simulink model "seldom_sim"  (R2024a)
settings: Solver=FixedStepAuto  StartTime=0.0  StopTime=30  FixedStep=framePeriod_s  RelTol=1e-9
values from neighbouring files (symbols this model uses):
  framePeriod_s = 1/frameRate_hz    (= 0.02)    [setup.m]
undefined symbols (not defined in the file or in its folder): accel_mps2, Aircraft, alt_wgs84_m, ch, current_ma, datetime, datevec, die_temp_c, Earth, Env, ext_gnss1, failsafe, fmu_imu, fmu_mag, frame_time_us, gps_tow_ms, gyro_radps, healthy, horz_acc_m, imu_healthy, inceptor, InitCond, installed, lat_rad, lon_rad, lost_frame, mag_ut, ned_vel_mps, new_data, num_sats, power_module, sys_time_us, Telem, vert_acc_m, voltage_v, week, WGS84
libraries: simulink x8, aerolibconvert2 x5, aerolibasang x3, aerolibtransform2 x2, aerolibgravity2 x2, aerolibatmos2 x1, sharedtransform x1, uavutilslib x1, vrlib x1, simulink_extras x1, spsLeadLagFilterLib x1, shared6dof x1
(part 1 of 2)
settings Model: SILPILSystemUnderTest=refmodels  Creator=brian  LastModifiedBy=joshb
settings SolverCC: AlgebraicLoopSolver=TrustRegion
settings DataIOCC: SaveOutput=off  SignalLogging=off  DSMLogging=off  SaveTime=off  ReturnWorkspaceOutputsName=Data
settings OptimizationCC: DefaultParameterBehavior=Inlined  EnhancedBackFolding=on  PassReuseOutputArgsAs=Individual arguments  ZeroExternalMemoryAtStartup=off  ZeroInternalMemoryAtStartup=off  OptimizeBlockOrder=speed  DifferentSizesBufferReuse=on  EfficientTunableParamExpr=on
settings DebuggingCC: Int32ToFloatConvMsg=none  ParameterPrecisionLossMsg=none  ParameterTunabilityLossMsg=error  UnconnectedInputMsg=warning  UnconnectedOutputMsg=warning  UnconnectedLineMsg=warning
settings HardwareCC: ProdBitPerPointer=32  ProdBitPerSizeT=32  ProdBitPerPtrDiffT=32  ProdLargestAtomicInteger=Long  ProdLargestAtomicFloat=Double  ProdWordSize=32  ProdHWDeviceType=NXP->Cortex-M4  TargetBitPerLong=64  TargetBitPerPointer=64  TargetBitPerSizeT=64  TargetBitPerPtrDiffT=64  TargetLargestAtomicFloat=Float  TargetIntDivRoundTo=Zero  TargetEndianess=LittleEndian  TargetWordSize=64  TargetHWDeviceType=Intel->x86-64 (Linux 64)  ProdEqTarget=off
settings ModelReferenceCC: UpdateModelReferenceTargets=Force  EnableRefExpFcnMdlSchedulingChecks=on
settings SFSimCC: SimCustomCompilerFlags=-std=c++2a, -fconcepts, -felide-constructors  SimCustomLinkerFlags=-std=c++2a, -fconcepts, -felide-constructors  MATLABDynamicMemAlloc=off  SimTargetLang=C++
settings RTWCC: Description=Embedded Coder  SystemTargetFile=ert.tlc  GenCodeOnly=on  TemplateMakefile=ert_default_tmf  RTWUseSimCustomCode=on  TargetLang=C++  GPUComputeCapability=3.5  DLArmComputeVersion=19.05
settings CodeAppCC: ForceParamTrailComments=on  IgnoreCustomStorageClasses=off  OperatorAnnotations=on  SimulinkDataObjDesc=on  SFDataObjDesc=on  InsertBlockDesc=on
settings ERTTargetCC: TargetLangStandard=C++11 (ISO)  GenerateSampleERTMain=on  CodeInterfacePackaging=C++ class  InlinedParameterPlacement=NonHierarchical  RootIOFormat=Structure reference  ERTCustomFileTemplate=example_file_process.tlc

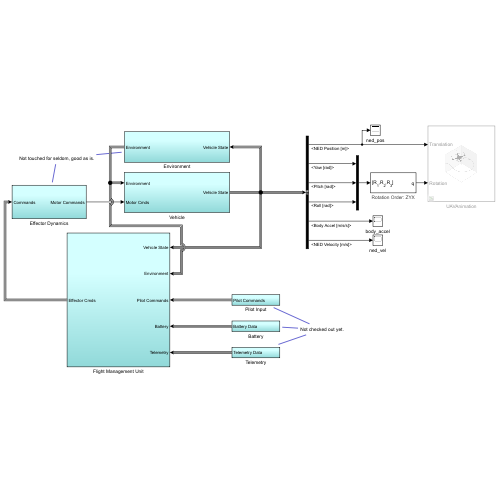
[thumbnail: Simulink's stored preview of the top-level diagram]
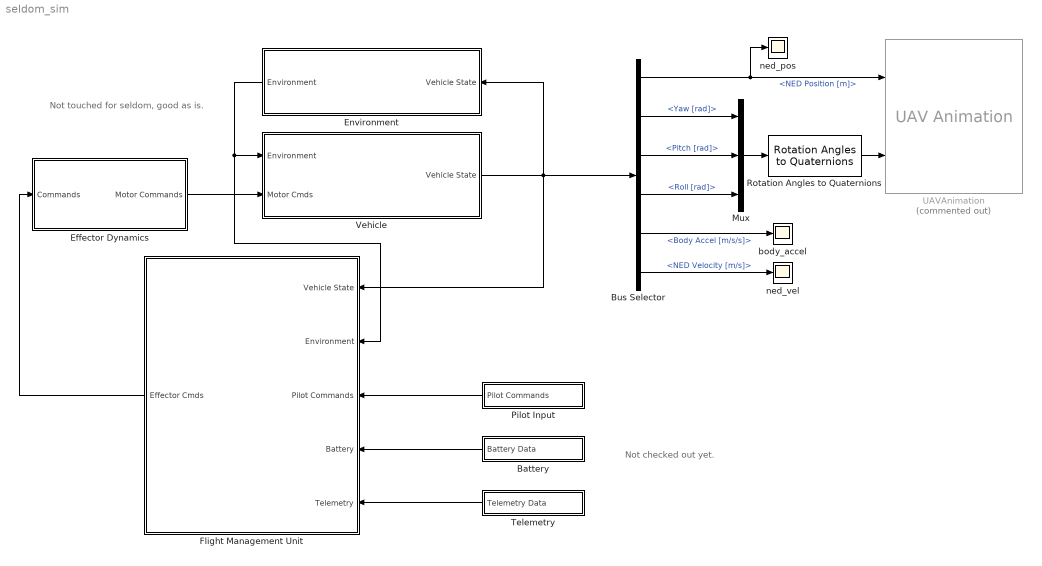
== system seldom_sim ==
  note: Not touched for seldom, good as is.
  note: Not checked out yet.
  Battery : Subsystem
  Bus Selector : BusSelector  OutputSignals=NED Position [m],Yaw [rad],Pitch [rad],Roll [rad],Body Accel [m/s/s],NED Velocity [m/s]
  Effector Dynamics : Subsystem
  Environment : Subsystem
  Flight Management Unit : Subsystem
  Mux : Mux  Inputs=3
  Pilot Input : Subsystem
  Rotation Angles to Quaternions : sharedtransform/Rotation Angles to Quaternions  rotationOrder=ZYX  aMode=aMode
  Telemetry : Subsystem
  UAVAnimation : uavutilslib/UAV Animation  Commented=on  UAVType=Multirotor  UAVSize=1  InertialZDirection=Down  SampleTime=-1
  Vehicle : Subsystem
  body_accel : Scope
  ned_pos : Scope
  ned_vel : Scope
  wires:
  Vehicle/1(Vehicle State) -> Environment/1(Vehicle State), Bus Selector/1, Flight Management Unit/1(Vehicle State)
  Pilot Input/1(Pilot Commands) -> Flight Management Unit/3(Pilot Commands)
  Environment/1(Environment) -> Vehicle/1(Environment), Flight Management Unit/2(Environment)
  Effector Dynamics/1(Motor Commands) -> Vehicle/2(Motor Cmds)
  Telemetry/1(Telemetry Data) -> Flight Management Unit/5(Telemetry)
  Flight Management Unit/1(Effector Cmds) -> Effector Dynamics/1(Commands)
  Battery/1(Battery Data) -> Flight Management Unit/4(Battery)
  Bus Selector/1 -> UAVAnimation/1, ned_pos/1  "<NED Position [m]>"
  Bus Selector/4 -> Mux/3  "<Roll [rad]>"
  Bus Selector/2 -> Mux/1  "<Yaw [rad]>"
  Bus Selector/3 -> Mux/2  "<Pitch [rad]>"
  Mux/1 -> Rotation Angles to Quaternions/1
  Rotation Angles to Quaternions/1 -> UAVAnimation/2
  Bus Selector/5 -> body_accel/1  "<Body Accel [m/s/s]>"
  Bus Selector/6 -> ned_vel/1  "<NED Velocity [m/s]>"

== system seldom_sim/Battery ==
  note: All of this needs updated for seldom. Or more likely it can all just go away, probably don't need it.
  note: This is the amp draw from the battery
  note: The mRo Power Zero module
      | outputs 1V for 33.594 amps drawn
      | from the battery
  note: This is the voltage measured by the FMU
      | power port. It is typically the current, scaled
      | by the power module mA / volt
  note: This is the voltage
      | measured by the FMU at
      | the power port. It is typically
      | the battery voltage scaled by the
      | power module voltage divider.
  note: The mRo Power Zero module
      | outputs 1V for 15.30 V at the
      | battery
  Bus Creator : BusCreator  Inputs=2
  Cast To Single : DataTypeConversion  OutDataTypeStr=single  SaturateOnIntegerOverflow=off  RndMeth=Floor
  Cast To Single1 : DataTypeConversion  OutDataTypeStr=single  SaturateOnIntegerOverflow=off  RndMeth=Floor
  Constant : Constant  Value=Aircraft.Battery.Voltage
  Constant1 : Constant  Value=42
  Constant2 : Constant
  Constant3 : Constant
  Divide : Product  Inputs=*/
  Divide1 : Product  Inputs=*/
  Battery Data : Outport
  wires:
  Bus Creator/1 -> Battery Data/1
  Constant2/1 -> Divide/2
  Constant1/1 -> Divide/1
  Divide/1 -> Cast To Single1/1  "Current [V]"
  Divide1/1 -> Cast To Single/1  "Voltage [V]"
  Constant/1 -> Divide1/1
  Constant3/1 -> Divide1/2
  Cast To Single/1 -> Bus Creator/1  "Voltage [V]"
  Cast To Single1/1 -> Bus Creator/2  "Current [V]"

== system seldom_sim/Effector Dynamics ==
  Commands : Inport
  Add1 : Sum
  Bus Selector : BusSelector  OutputSignals=pwm
  Constant : Constant  Value=0
  Constant1 : Constant  Commented=on  Value=InitCond.motor_cmd
  Selector1 : Selector  InputPortWidth=Aircraft.Eff.nPwm  IndexOptions=Index vector (dialog)  Indices=Aircraft.Motor.map  OutputSizes=1
  Motor Commands : Outport
  wires:
  Constant/1 -> Add1/2
  Selector1/1 -> Add1/1
  Bus Selector/1 -> Selector1/1  "<pwm>"
  Commands/1 -> Bus Selector/1
  Add1/1 -> Motor Commands/1

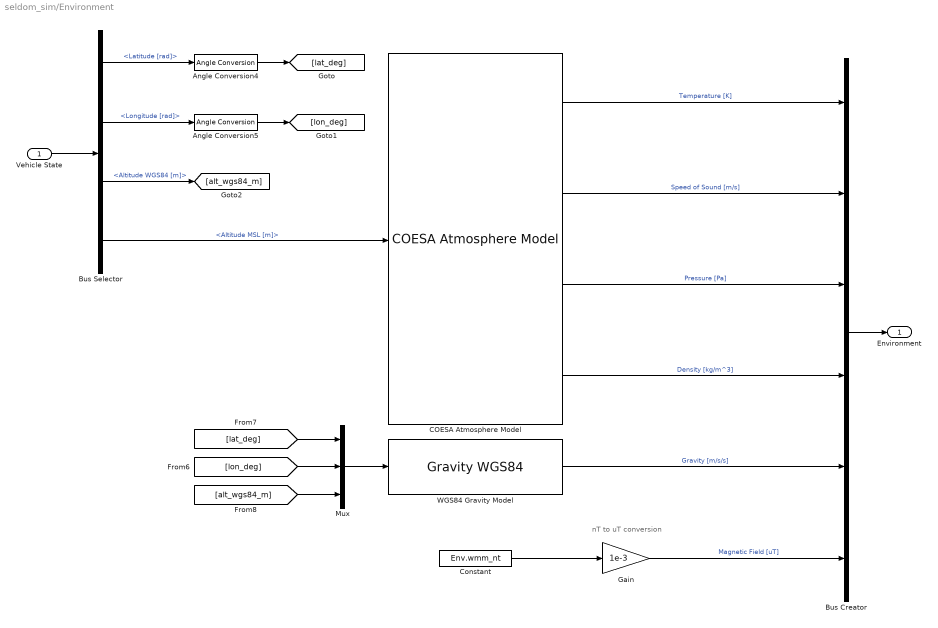
== system seldom_sim/Environment ==
  note: nT to uT conversion
  Vehicle State : Inport
  Angle Conversion4 : aerolibconvert2/Angle Conversion  IU=rad  OU=deg
  Angle Conversion5 : aerolibconvert2/Angle Conversion  IU=rad  OU=deg
  Bus Creator : BusCreator  Inputs=6
  Bus Selector : BusSelector  OutputSignals=Latitude [rad],Longitude [rad],Altitude WGS84 [m],Altitude MSL [m]
  COESA Atmosphere Model : aerolibatmos2/COESA Atmosphere Model  units=Metric (MKS)  spec=1976 COESA-extended U.S. Standard Atmosphere  model=Profile  profile_var=High temperature  profile_percent=1%  profile_alt=5 km (16404 ft)  envelope_var=High temperature  envelope_percent=1%  action=Warning
  Constant : Constant  Value=Env.wmm_nt
  Gain : Gain  Gain=1e-3
  Mux : Mux  Inputs=3
  "WGS84 Gravity Model  " : GravityWGS84
  Environment : Outport
  wires:
  [lon_deg] -> Mux/2
  COESA Atmosphere Model/4 -> Bus Creator/4  "Density [kg/m^3]"
  Mux/1 -> "WGS84 Gravity Model  "/1
  Bus Selector/3 -> [alt_wgs84_m]  "<Altitude WGS84 [m]>"
  Vehicle State/1 -> Bus Selector/1
  Bus Selector/2 -> Angle Conversion5/1  "<Longitude [rad]>"
  COESA Atmosphere Model/2 -> Bus Creator/2  "Speed of Sound [m/s]"
  Bus Selector/4 -> COESA Atmosphere Model/1  "<Altitude MSL [m]>"
  [alt_wgs84_m] -> Mux/3
  Angle Conversion4/1 -> [lat_deg]
  [lat_deg] -> Mux/1
  Bus Creator/1 -> Environment/1
  Constant/1 -> Gain/1
  Gain/1 -> Bus Creator/6  "Magnetic Field [uT]"
  "WGS84 Gravity Model  "/1 -> Bus Creator/5  "Gravity [m/s/s]"
  Bus Selector/1 -> Angle Conversion4/1  "<Latitude [rad]>"
  COESA Atmosphere Model/3 -> Bus Creator/3  "Pressure [Pa]"
  COESA Atmosphere Model/1 -> Bus Creator/1  "Temperature [K]"
  Angle Conversion5/1 -> [lon_deg]

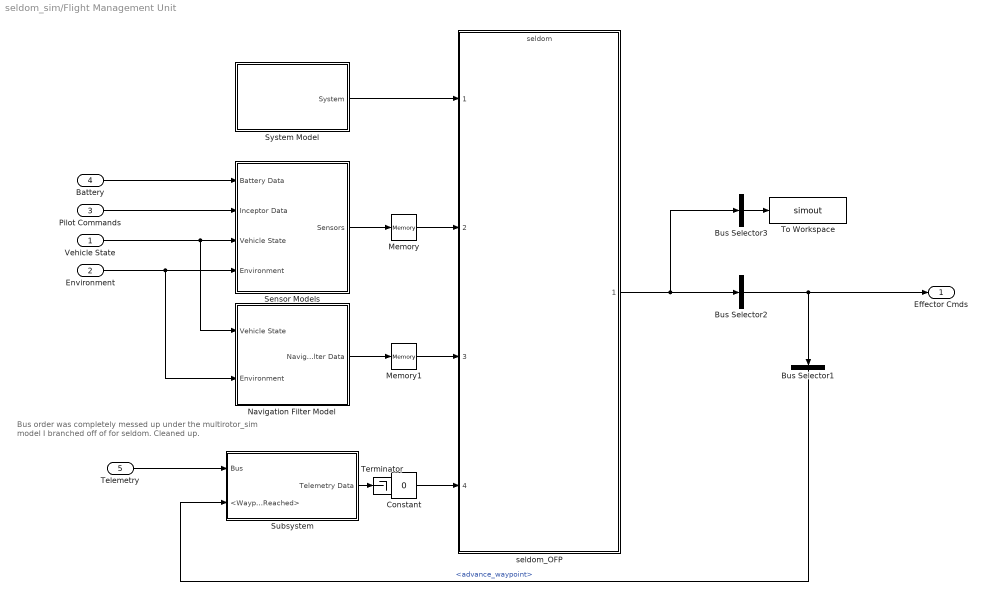
== system seldom_sim/Flight Management Unit ==
  note: Bus order was completely messed up under the multirotor_sim model I branched off of for seldom. Cleaned up.
  Vehicle State : Inport
  Environment : Inport  Port=2
  Pilot Commands : Inport  Port=3
  Battery : Inport  Port=4
  Telemetry : Inport  Port=5
  Bus Selector1 : BusSelector  OutputSignals=advance_waypoint
  Bus Selector2 : BusSelector  OutputSignals=advance_waypoint,sbus,pwm  OutputAsBus=on
  Bus Selector3 : BusSelector  OutputSignals=aux  OutputAsBus=on
  Constant : Constant  Value=0  OutDataTypeStr=Bus: TelemData
  Memory : Memory  InheritSampleTime=on  LinearizeMemory=on  LinearizeAsDelay=on
  Memory1 : Memory  InheritSampleTime=on  LinearizeMemory=on  LinearizeAsDelay=on
  Navigation Filter Model : Subsystem
      settings: PortSchema="{\"entries\":[{\"content\":{\"sides\":[{\"content\":{\"connectorIds\":[]},\"type\":\"ConnectorPlacement.EquallySpacedRectSide\",\"uuid\":\"b20f7590-d69b-48b8-beb1-2fb7d3ab0357\"},{\"content\":{\"connectorIds\":[],\"side\":\"RIGHT\"},\"type\":\"ConnectorPlacement.EquallySpacedRectSide\",\"uuid\":\"07801f8a-7756-483e-a050-3c2fccc33404\"},{\"content\":{\"connectorIds\":[\"In1\",\"In2\"],\"side\":\"TOP\"},\"type\":\"ConnectorPlacement.EquallySpacedRectSide\",\"uuid\":\"ce3c3c94-ed36-4103-b079-69dcaeaf21e9\"},{\"content\":{\"connectorIds\":[\"Out1\"],\"side\":\"BOTTOM\"},\"type\":\"ConnectorPlacement.EquallySpacedRectSide\",\"uuid\":\"ba78b819-a471-4bc3-b479-e6a973cfe14f\"},{\"content\":{\"connectorIds\":[],\"side\":\"HIDDEN\"},\"type\":\"ConnectorPlacement.EquallySpacedRectSide\",\"uuid\":\"3cf915a5-25a1-4380-9090-9561533312da\"}]},\"type\":\"ConnectorPlacement.EquallySpacedConnector\",\"uuid\":\"7ef4ddaa-ccd2-4778-89ce-8b4685524e82\"}],\"packageUris\":[\"http://schema.mathworks.com/mf0/Connector/R2020b\"],\"version\":\"1.0\"}"
  Sensor Models : Subsystem
      settings: PortSchema="{\"entries\":[{\"content\":{\"sides\":[{\"content\":{},\"type\":\"ConnectorPlacement.EquallySpacedRectSide\",\"uuid\":\"b20f7590-d69b-48b8-beb1-2fb7d3ab0357\"},{\"content\":{\"side\":\"RIGHT\"},\"type\":\"ConnectorPlacement.EquallySpacedRectSide\",\"uuid\":\"07801f8a-7756-483e-a050-3c2fccc33404\"},{\"content\":{\"connectorIds\":[\"In1\",\"In2\",\"In3\",\"In4\"],\"side\":\"TOP\"},\"type\":\"ConnectorPlacement.EquallySpacedRectSide\",\"uuid\":\"ce3c3c94-ed36-4103-b079-69dcaeaf21e9\"},{\"content\":{\"connectorIds\":[\"Out1\"],\"side\":\"BOTTOM\"},\"type\":\"ConnectorPlacement.EquallySpacedRectSide\",\"uuid\":\"ba78b819-a471-4bc3-b479-e6a973cfe14f\"},{\"content\":{\"side\":\"HIDDEN\"},\"type\":\"ConnectorPlacement.EquallySpacedRectSide\",\"uuid\":\"3cf915a5-25a1-4380-9090-9561533312da\"}]},\"type\":\"ConnectorPlacement.EquallySpacedConnector\",\"uuid\":\"7ef4ddaa-ccd2-4778-89ce-8b4685524e82\"}],\"packageUris\":[\"http://schema.mathworks.com/mf0/Connector/R2020b\"],\"version\":\"1.0\"}"
  Subsystem : Subsystem
  System Model : Subsystem
      settings: PortSchema="{\"entries\":[{\"content\":{\"sides\":[{\"content\":{\"connectorIds\":[]},\"type\":\"ConnectorPlacement.EquallySpacedRectSide\",\"uuid\":\"b20f7590-d69b-48b8-beb1-2fb7d3ab0357\"},{\"content\":{\"connectorIds\":[],\"side\":\"RIGHT\"},\"type\":\"ConnectorPlacement.EquallySpacedRectSide\",\"uuid\":\"07801f8a-7756-483e-a050-3c2fccc33404\"},{\"content\":{\"connectorIds\":[],\"side\":\"TOP\"},\"type\":\"ConnectorPlacement.EquallySpacedRectSide\",\"uuid\":\"ce3c3c94-ed36-4103-b079-69dcaeaf21e9\"},{\"content\":{\"connectorIds\":[\"Out1\"],\"side\":\"BOTTOM\"},\"type\":\"ConnectorPlacement.EquallySpacedRectSide\",\"uuid\":\"ba78b819-a471-4bc3-b479-e6a973cfe14f\"},{\"content\":{\"connectorIds\":[],\"side\":\"HIDDEN\"},\"type\":\"ConnectorPlacement.EquallySpacedRectSide\",\"uuid\":\"3cf915a5-25a1-4380-9090-9561533312da\"}]},\"type\":\"ConnectorPlacement.EquallySpacedConnector\",\"uuid\":\"7ef4ddaa-ccd2-4778-89ce-8b4685524e82\"}],\"packageUris\":[\"http://schema.mathworks.com/mf0/Connector/R2020b\"],\"version\":\"1.0\"}"
  Terminator : Terminator
  To Workspace : ToWorkspace  VariableName=simout  SaveFormat=Timeseries  SampleTime=-1
  seldom_OFP : ModelReference  ModelNameDialog=seldom.slx  SimulationMode=Normal  ModelReferenceVersion=8.65
  Effector Cmds : Outport
  wires:
  Environment/1 -> Navigation Filter Model/1(Environment), Sensor Models/1(Environment)
  Vehicle State/1 -> Navigation Filter Model/2(Vehicle State), Sensor Models/2(Vehicle State)
  Sensor Models/1(Sensors) -> Memory/1
  Navigation Filter Model/1(Navigation Filter Data) -> Memory1/1
  System Model/1(System) -> seldom_OFP/1
  Pilot Commands/1 -> Sensor Models/3(Inceptor Data)
  Telemetry/1 -> Subsystem/1(Bus)
  Memory/1 -> seldom_OFP/2
  Memory1/1 -> seldom_OFP/3
  Battery/1 -> Sensor Models/4(Battery Data)
  Subsystem/1(Telemetry Data) -> Terminator/1
  Bus Selector1/1 -> Subsystem/2(<Waypoint Reached>)  "<advance_waypoint>"
  Bus Selector2/1 -> Bus Selector1/1, Effector Cmds/1
  seldom_OFP/1 -> Bus Selector3/1, Bus Selector2/1
  Constant/1 -> seldom_OFP/4
  Bus Selector3/1 -> To Workspace/1

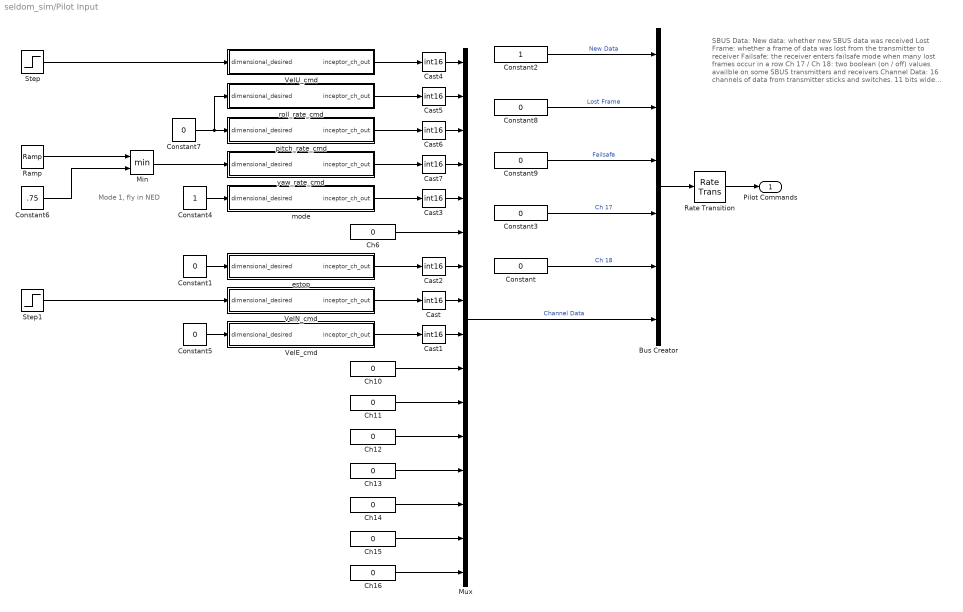
== system seldom_sim/Pilot Input ==
  note: Mode 1, fly in NED
  note: SBUS Data:
      | New data: whether new SBUS data was received
      | Lost Frame: whether a frame of data was lost from the transmitter to receiver
      | Failsafe: the receiver enters failsafe mode when many lost frames occur in a row
      | Ch 17 / Ch 18: two boolean (on / off) values availble on some SBUS transmitters and receivers
      | Channel Data: 16 channels of data from transmitter sticks and switches. 11 bits wide limiting values to 0 - 2048. Actual ranges may be different, for example, FrSky typically uses 172 - 1811 unless its range is extended to +/- 150%
  Bus Creator : BusCreator  Inputs=6
  Cast{,1..7} (8 alike) : DataTypeConversion  OutDataTypeStr=int16  SaturateOnIntegerOverflow=off  RndMeth=Floor
  Ch{6,10..16} (8 alike) : Constant  Value=0  OutDataTypeStr=int16
  Constant : Constant  Value=0  OutDataTypeStr=int8
  Constant1 : Constant  Value=0
  Constant2 : Constant  OutDataTypeStr=boolean
  Constant3 : Constant  Value=0  OutDataTypeStr=boolean
  Constant4 : Constant
  Constant5 : Constant  Value=0
  Constant6 : Constant  Value=.75
  Constant7 : Constant  Value=0
  Constant8 : Constant  Value=0  OutDataTypeStr=boolean
  Constant9 : Constant  Value=0  OutDataTypeStr=boolean
  Min : MinMax  Inputs=2
  Mux : Mux  Inputs=16
  Ramp : simulink/Sources/Ramp  slope=0.25  start=22  InitialOutput=0
  Rate Transition : RateTransition  OutPortSampleTime=framePeriod_s
  Step : Step  After=2  SampleTime=0
  Step1 : Step  Time=8  SampleTime=0
  VelE_cmd : Subsystem
  VelN_cmd : Subsystem
  VelU_cmd : Subsystem
  estop : Subsystem
  mode : Subsystem
  pitch_rate_cmd : Subsystem
  roll_rate_cmd : Subsystem
  yaw_rate_cmd : Subsystem
  Pilot Commands : Outport
  wires:
  Bus Creator/1 -> Rate Transition/1
  Constant2/1 -> Bus Creator/1  "New Data"
  Constant8/1 -> Bus Creator/2  "Lost Frame"
  Constant9/1 -> Bus Creator/3  "Failsafe"
  Constant3/1 -> Bus Creator/4  "Ch 17"
  Constant/1 -> Bus Creator/5  "Ch 18"
  Mux/1 -> Bus Creator/6  "Channel Data"
  VelU_cmd/1(inceptor_ch_out) -> Cast4/1
  Ch16/1 -> Mux/16
  Ch15/1 -> Mux/15
  Ch14/1 -> Mux/14
  Ch13/1 -> Mux/13
  Ch12/1 -> Mux/12
  Ch11/1 -> Mux/11
  Ch10/1 -> Mux/10
  VelE_cmd/1(inceptor_ch_out) -> Cast1/1
  VelN_cmd/1(inceptor_ch_out) -> Cast/1
  estop/1(inceptor_ch_out) -> Cast2/1
  Ch6/1 -> Mux/6
  yaw_rate_cmd/1(inceptor_ch_out) -> Cast7/1
  roll_rate_cmd/1(inceptor_ch_out) -> Cast5/1
  pitch_rate_cmd/1(inceptor_ch_out) -> Cast6/1
  mode/1(inceptor_ch_out) -> Cast3/1
  Cast/1 -> Mux/8
  Cast1/1 -> Mux/9
  Constant1/1 -> estop/1(dimensional_desired)
  Cast2/1 -> Mux/7
  Constant4/1 -> mode/1(dimensional_desired)
  Cast3/1 -> Mux/5
  Cast4/1 -> Mux/1
  Cast5/1 -> Mux/2
  Cast6/1 -> Mux/3
  Cast7/1 -> Mux/4
  Step/1 -> VelU_cmd/1(dimensional_desired)
  Step1/1 -> VelN_cmd/1(dimensional_desired)
  Constant5/1 -> VelE_cmd/1(dimensional_desired)
  Ramp/1 -> Min/1
  Constant6/1 -> Min/2
  Min/1 -> yaw_rate_cmd/1(dimensional_desired)
  Constant7/1 -> roll_rate_cmd/1(dimensional_desired), pitch_rate_cmd/1(dimensional_desired)
  Rate Transition/1 -> Pilot Commands/1

== system seldom_sim/Telemetry ==
  Bus Creator : BusCreator  Inputs=11
  Constant1 : Constant  Value=0  OutDataTypeStr=boolean
  Constant10 : Constant  Value=Telem.Fence  OutDataTypeStr=Bus: MissionItem
  Constant11 : Constant  Value=Telem.Rally  OutDataTypeStr=Bus: MissionItem
  Constant2 : Constant  Value=0  OutDataTypeStr=boolean
  Constant3 : Constant  OutDataTypeStr=int16
  Constant4 : Constant  Value=0  OutDataTypeStr=int16
  Constant5 : Constant  Value=0  OutDataTypeStr=int16
  Constant6 : Constant  Value=0  OutDataTypeStr=int16
  Constant7 : Constant  Value=[0 0 0 0 0 0 0 0 0 1 1 1 1 0 0 0 0 0 0 0 0 0 0 0]  OutDataTypeStr=boolean
  Constant8 : Constant  Value=0  OutDataTypeStr=boolean
  Constant9 : Constant  Value=Telem.FlightPlan  OutDataTypeStr=Bus: MissionItem
  Telemetry Data : Outport
  wires:
  Bus Creator/1 -> Telemetry Data/1
  Constant8/1 -> Bus Creator/1  "Waypoints Updated"
  Constant1/1 -> Bus Creator/2  "Fence Updated"
  Constant2/1 -> Bus Creator/3  "Rally Points Updated"
  Constant3/1 -> Bus Creator/4  "Current Waypoint Index"
  Constant4/1 -> Bus Creator/5  "Number of Waypoints"
  Constant5/1 -> Bus Creator/6  "Number of Fence Points"
  Constant6/1 -> Bus Creator/7  "Number of Rally Points"
  Constant7/1 -> Bus Creator/8  "Parameters"
  Constant9/1 -> Bus Creator/9  "Flight Plan"
  Constant10/1 -> Bus Creator/10  "Fence"
  Constant11/1 -> Bus Creator/11  "Rally"

== system seldom_sim/Vehicle ==
  note: Not touched for seldom, good as is.
  Environment : Inport
  Motor Cmds : Inport  Port=2
  Bus Creator : BusCreator  Inputs=26
  Bus Selector : BusSelector  OutputSignals=Gravity [m/s/s],Density [kg/m^3],Speed of Sound [m/s]
  Bus Selector1 : BusSelector  OutputSignals=Dynamic Pressure [Pa],DCM_be,Body Velocity [m/s]
  Forces and Moments : Subsystem
  Vehicle Model : Subsystem
  Vehicle State : Outport
  wires:
  Bus Selector/1 -> Forces and Moments/5(Gravity [m/s/s])  "<Gravity [m/s/s]>"
  Vehicle Model/20(Angle of Attack Rate [rad/s]) -> Bus Creator/20  "Angle of Attack Rate [rad/s]"
  Bus Selector1/1 -> Forces and Moments/1(Dynamic Pressure [Pa])  "<Dynamic Pressure [Pa]>"
  Vehicle Model/4(Altitude MSL [m]) -> Bus Creator/4  "Altitude MSL [m]"
  Vehicle Model/26(DCM_be) -> Bus Creator/26  "DCM_be"
  Vehicle Model/16(Dynamic Pressure [Pa]) -> Bus Creator/16  "Dynamic Pressure [Pa]"
  Vehicle Model/22(Sideslip Angle Rate [rad/s]) -> Bus Creator/22  "Sideslip Angle Rate [rad/s]"
  Vehicle Model/21(Sideslip Angle [rad]) -> Bus Creator/21  "Sideslip Angle [rad]"
  Vehicle Model/24(Flight Path Angle [rad]) -> Bus Creator/24  "Flight Path Angle [rad]"
  Vehicle Model/11(Yaw [rad]) -> Bus Creator/11  "Yaw [rad]"
  Vehicle Model/18(Mach) -> Bus Creator/18  "Mach"
  Vehicle Model/5(Altitude AGL [m]) -> Bus Creator/5  "Altitude AGL [m]"
  Bus Selector1/2 -> Forces and Moments/2(DCM_be)  "<DCM_be>"
  Bus Selector/2 -> Vehicle Model/3(Density [kg/m^3])  "<Density [kg/m^3]>"
  Vehicle Model/6(NED Position [m]) -> Bus Creator/6  "NED Position [m]"
  Vehicle Model/23(Ground Track [rad]) -> Bus Creator/23  "Ground Track [rad]"
  Vehicle Model/10(Roll [rad]) -> Bus Creator/10  "Roll [rad]"
  Vehicle Model/7(NED Velocity [m/s]) -> Bus Creator/7  "NED Velocity [m/s]"
  Vehicle Model/17(Airspeed [m/s]) -> Bus Creator/17  "Airspeed [m/s]"
  Vehicle Model/15(Body Rotational Accel [rad/s/s]) -> Bus Creator/15  "Body Rotational Accel [rad/s/s]"
  Vehicle Model/14(Body Rotational Rate [rad/s]) -> Bus Creator/14  "Body Rotational Rate [rad/s]"
  Vehicle Model/13(Body Accel [m/s/s]) -> Bus Creator/13  "Body Accel [m/s/s]"
  Vehicle Model/9(Pitch [rad]) -> Bus Creator/9  "Pitch [rad]"
  Vehicle Model/8(NED Accel [m/s/s]) -> Bus Creator/8  "NED Accel [m/s/s]"
  Forces and Moments/2(Mxyz [N-m]) -> Vehicle Model/2(Mxyz [N-m])
  Environment/1 -> Bus Selector/1
  Bus Selector/3 -> Vehicle Model/4(Speed of Sound [m/s])  "<Speed of Sound [m/s]>"
  Bus Creator/1 -> Bus Selector1/1, Vehicle State/1
  Forces and Moments/1(Fxyz [N]) -> Vehicle Model/1(Fxyz [N])
  Vehicle Model/19(Angle of Attack [rad]) -> Bus Creator/19  "Angle of Attack [rad]"
  Vehicle Model/3(Altitude WGS84 [m]) -> Bus Creator/3  "Altitude WGS84 [m]"
  Motor Cmds/1 -> Forces and Moments/4(Motor Cmds)
  Vehicle Model/2(Longitude [rad]) -> Bus Creator/2  "Longitude [rad]"
  Vehicle Model/1(Latitude [rad]) -> Bus Creator/1  "Latitude [rad]"
  Vehicle Model/12(Body Velocity [m/s]) -> Bus Creator/12  "Body Velocity [m/s]"
  Vehicle Model/25(Ground Speed [m/s]) -> Bus Creator/25  "Ground Speed [m/s]"
  Bus Selector1/3 -> Forces and Moments/3(body_vel)  "<Body Velocity [m/s]>"

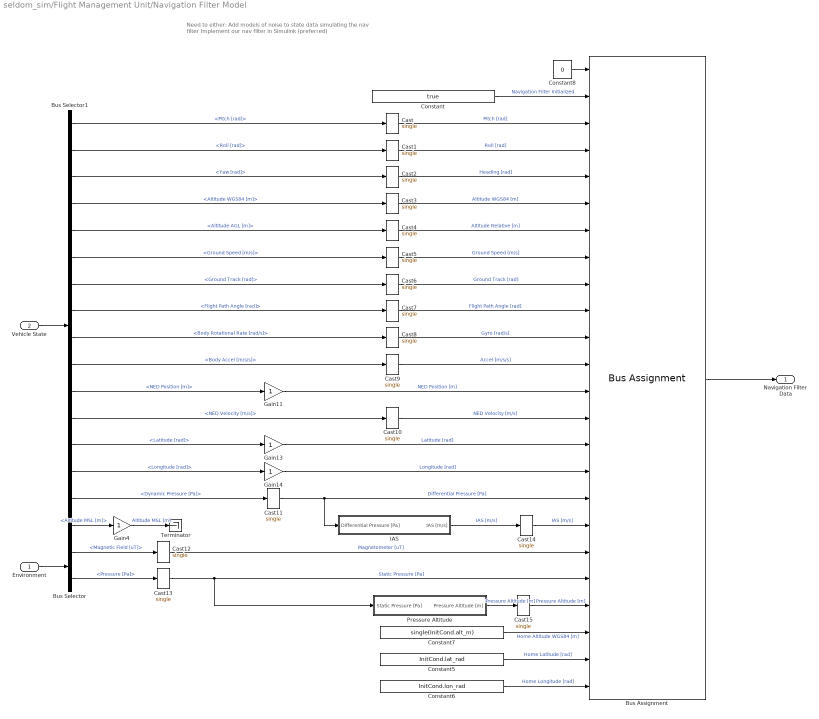
== system seldom_sim/Flight Management Unit/Navigation Filter Model ==
  note: Need to either:
      | Add models of noise to state data simulating the nav filter
      | Implement our nav filter in Simulink (preferred)
  Environment : Inport
  Vehicle State : Inport  Port=2
  Bus Assignment : BusAssignment  AssignedSignals=bfs_ins.initialized,bfs_ins.pitch_rad,bfs_ins.roll_rad,bfs_ins.heading_rad,bfs_ins.alt_wgs84_m,adc.rel_alt_m,aux_ins.gnd_spd_mps,aux_ins.gnd_track_rad,aux_ins.flight_path_rad,bfs_ins.gyro_radps,bfs_ins.accel_mps2,aux_ins.ned_pos_m,bfs_ins.ned_vel_mps,bfs_ins.lat_rad,bfs_ins.lon_rad,adc.diff_press_pa,adc.ias_mps,bfs_ins.mag_ut,adc.static_pres_pa,adc.pres_alt_m,aux_ins.home_alt_wgs84_m,aux_ins.home_lat_rad,aux_ins.home_lon_rad
  Bus Selector : BusSelector  OutputSignals=Magnetic Field [uT],Pressure [Pa]
  Bus Selector1 : BusSelector  OutputSignals=Pitch [rad],Roll [rad],Yaw [rad],Altitude WGS84 [m],Altitude AGL [m],Ground Speed [m/s],Ground Track [rad],Flight Path Angle [rad],Body Rotational Rate [rad/s],Body Accel [m/s/s],NED Position [m],NED Velocity [m/s],Latitude [rad],Longitude [rad],Dynamic Pressure [Pa],Altitude MSL [m]
  Cast{,1..15} (16 alike) : DataTypeConversion  OutDataTypeStr=single  SaturateOnIntegerOverflow=off  RndMeth=Floor
  Constant : Constant  Value=true
  Constant5 : Constant  Value=InitCond.lat_rad
  Constant6 : Constant  Value=InitCond.lon_rad
  Constant7 : Constant  Value=single(InitCond.alt_m)
  Constant8 : Constant  Value=0  OutDataTypeStr=Bus: StateEstData
  Gain{4,11,13..14} (4 alike) : Gain
  IAS : Subsystem
  Pressure Altitude : Subsystem
  Terminator : Terminator
  Navigation Filter Data : Outport
  wires:
  Environment/1 -> Bus Selector/1
  Bus Assignment/1 -> Navigation Filter Data/1
  Vehicle State/1 -> Bus Selector1/1
  Constant/1 -> Bus Assignment/2  "Navigation Filter Initialized"
  Bus Selector1/1 -> Cast/1  "<Pitch [rad]>"
  Bus Selector1/2 -> Cast1/1  "<Roll [rad]>"
  Bus Selector1/3 -> Cast2/1  "<Yaw [rad]>"
  Bus Selector1/4 -> Cast3/1  "<Altitude WGS84 [m]>"
  Bus Selector1/16 -> Gain4/1  "<Altitude MSL [m]>"
  Bus Selector1/5 -> Cast4/1  "<Altitude AGL [m]>"
  Bus Selector1/6 -> Cast5/1  "<Ground Speed [m/s]>"
  Bus Selector1/7 -> Cast6/1  "<Ground Track [rad]>"
  Bus Selector1/8 -> Cast7/1  "<Flight Path Angle [rad]>"
  Bus Selector1/9 -> Cast8/1  "<Body Rotational Rate [rad/s]>"
  Bus Selector1/10 -> Cast9/1  "<Body Accel [m/s/s]>"
  Bus Selector1/11 -> Gain11/1  "<NED Position [m]>"
  Bus Selector1/12 -> Cast10/1  "<NED Velocity [m/s]>"
  Bus Selector/2 -> Cast13/1  "<Pressure [Pa]>"
  Pressure Altitude/1(Pressure Altitude [m]) -> Cast15/1  "Pressure Altitude [m]"
  Bus Selector/1 -> Cast12/1  "<Magnetic Field [uT]>"
  IAS/1(IAS [m/s]) -> Cast14/1  "IAS [m/s]"
  Bus Selector1/15 -> Cast11/1  "<Dynamic Pressure [Pa]>"
  Bus Selector1/14 -> Gain14/1  "<Longitude [rad]>"
  Bus Selector1/13 -> Gain13/1  "<Latitude [rad]>"
  Cast/1 -> Bus Assignment/3  "Pitch [rad]"
  Cast1/1 -> Bus Assignment/4  "Roll [rad]"
  Cast2/1 -> Bus Assignment/5  "Heading [rad]"
  Cast3/1 -> Bus Assignment/6  "Altitude WGS84 [m]"
  Gain4/1 -> Terminator/1  "Altitude MSL [m]"
  Cast4/1 -> Bus Assignment/7  "Altitude Relative [m]"
  Cast5/1 -> Bus Assignment/8  "Ground Speed [m/s]"
  Cast6/1 -> Bus Assignment/9  "Ground Track [rad]"
  Cast7/1 -> Bus Assignment/10  "Flight Path Angle [rad]"
  Cast8/1 -> Bus Assignment/11  "Gyro [rad/s]"
  Cast9/1 -> Bus Assignment/12  "Accel [m/s/s]"
  Gain11/1 -> Bus Assignment/13  "NED Position [m]"
  Cast10/1 -> Bus Assignment/14  "NED Velocity [m/s]"
  Gain13/1 -> Bus Assignment/15  "Latitude [rad]"
  Gain14/1 -> Bus Assignment/16  "Longitude [rad]"
  Cast11/1 -> Bus Assignment/17, IAS/1(Differential Pressure [Pa])  "Differential Pressure [Pa]"
  Cast12/1 -> Bus Assignment/19  "Magnetometer [uT]"
  Cast13/1 -> Pressure Altitude/1(Static Pressure [Pa]), Bus Assignment/20  "Static Pressure [Pa]"
  Constant5/1 -> Bus Assignment/23  "Home Latitude [rad]"
  Constant6/1 -> Bus Assignment/24  "Home Longitude [rad]"
  Constant7/1 -> Bus Assignment/22  "Home Altitude WGS84 [m]"
  Constant8/1 -> Bus Assignment/1
  Cast14/1 -> Bus Assignment/18  "IAS [m/s]"
  Cast15/1 -> Bus Assignment/21  "Pressure Altitude [m]"

== system seldom_sim/Flight Management Unit/Sensor Models ==
  Environment : Inport
  Vehicle State : Inport  Port=2
  Inceptor Data : Inport  Port=3
  Battery Data : Inport  Port=4
  Bus Assignment : BusAssignment  AssignedSignals=inceptor,fmu_imu,fmu_mag,ext_gnss1,power_module
  Bus Selector : BusSelector  OutputSignals=Body Rotational Rate [rad/s],Body Accel [m/s/s],DCM_be
  Bus Selector1 : BusSelector  OutputSignals=Latitude [rad],Longitude [rad],Altitude WGS84 [m],NED Velocity [m/s]
  Bus Selector3 : BusSelector  OutputSignals=Gravity [m/s/s],Magnetic Field [uT]
  Constant5 : Constant  Value=0  OutDataTypeStr=Bus: SensorData
  GNSS : Subsystem
  IMU : Subsystem
  MakeInceptorBus : Subsystem
  MakePowerModuleBus : Subsystem
  Sensors : Outport
  wires:
  Bus Assignment/1 -> Sensors/1
  Vehicle State/1 -> Bus Selector1/1, Bus Selector/1
  Bus Selector/1 -> IMU/1(Body Rotational Rate [rad/s])  "<Body Rotational Rate [rad/s]>"
  Bus Selector/2 -> IMU/2(Body Accel [m/s/s])  "<Body Accel [m/s/s]>"
  Bus Selector/3 -> IMU/3(DCM_be)  "<DCM_be>"
  Bus Selector1/1 -> GNSS/1(Latitude [rad])  "<Latitude [rad]>"
  Bus Selector1/2 -> GNSS/2("Longitude [rad] ")  "<Longitude [rad]>"
  Bus Selector1/3 -> GNSS/3(Altitude WGS84 [m])  "<Altitude WGS84 [m]>"
  Bus Selector1/4 -> GNSS/4(NED Velocity [m/s])  "<NED Velocity [m/s]>"
  Environment/1 -> Bus Selector3/1
  Bus Selector3/1 -> IMU/4(Gravity [m/s/s])  "<Gravity [m/s/s]>"
  Bus Selector3/2 -> IMU/5(Magnetic Field [uT])  "<Magnetic Field [uT]>"
  IMU/1(IMUBus) -> Bus Assignment/3  "IMU"
  GNSS/1(GNSS Data) -> Bus Assignment/5  "GNSS"
  Battery Data/1 -> MakePowerModuleBus/1(Battery)  "Battery"
  Constant5/1 -> Bus Assignment/1
  Inceptor Data/1 -> MakeInceptorBus/1(Inceptor)  "Inceptor"
  MakeInceptorBus/1(InceptorBus) -> Bus Assignment/2
  MakePowerModuleBus/1(PowerModuleBus) -> Bus Assignment/6
  IMU/2(MagBus) -> Bus Assignment/4

== system seldom_sim/Flight Management Unit/Subsystem ==
  Bus : Inport
  <Waypoint Reached> : Inport  Port=2
  Bus Creator : BusCreator  Inputs=11
  Bus Selector1 : BusSelector  OutputSignals=Waypoints Updated,Fence Updated,Rally Points Updated,Current Waypoint Index,Number of Waypoints,Number of Fence Points,Number of Rally Points,Parameters,Flight Plan,Fence,Rally
  Terminator : Terminator
  Triggered Subsystem : Subsystem  TreatAsAtomicUnit=on
  Unit Delay : UnitDelay  SampleTime=-1  HasFrameUpgradeWarning=on
  Unit Delay1 : UnitDelay  SampleTime=-1  HasFrameUpgradeWarning=on
  Telemetry Data : Outport
  wires:
  Bus Selector1/9 -> Bus Creator/9  "<Flight Plan>"
  Bus Selector1/3 -> Bus Creator/3  "<Rally Points Updated>"
  Bus Selector1/6 -> Bus Creator/6  "<Number of Fence Points>"
  <Waypoint Reached>/1 -> Unit Delay1/1
  Bus Selector1/11 -> Bus Creator/11  "<Rally>"
  Bus Selector1/10 -> Bus Creator/10  "<Fence>"
  Bus Selector1/4 -> Terminator/1  "<Current Waypoint Index>"
  Bus Selector1/8 -> Bus Creator/8  "<Parameters>"
  Bus Selector1/7 -> Bus Creator/7  "<Number of Rally Points>"
  Bus Selector1/2 -> Bus Creator/2  "<Fence Updated>"
  Bus Selector1/5 -> Bus Creator/5  "<Number of Waypoints>"
  Bus Selector1/1 -> Bus Creator/1  "<Waypoints Updated>"
  Triggered Subsystem/1(Wp++) -> Bus Creator/4, Unit Delay/1  "Current Waypoint Index"
  Bus/1 -> Bus Selector1/1
  Bus Creator/1 -> Telemetry Data/1
  Unit Delay/1 -> Triggered Subsystem/1(Wp)
  Unit Delay1/1 -> Triggered Subsystem/Trigger

== system seldom_sim/Flight Management Unit/System Model ==
  note: Uses an integer since it is in microseconds.
  Bus Assignment : BusAssignment  AssignedSignals=frame_time_us,sys_time_us
  Cast : DataTypeConversion  OutDataTypeStr=int32  SaturateOnIntegerOverflow=off  RndMeth=Floor
  Cast1 : DataTypeConversion  OutDataTypeStr=int64  SaturateOnIntegerOverflow=off  RndMeth=Floor
  Clock : Clock
      settings: Decimation=1e6
  Constant4 : Constant  Value=framePeriod_s
  Constant5 : Constant  Value=0  OutDataTypeStr=Bus: SysData
  Gain : Gain  Gain=1e6
  Gain1 : Gain  Gain=1e6
  System : Outport
  wires:
  Clock/1 -> Gain/1  "System Time [s]"
  Constant4/1 -> Gain1/1  "Frame Time [s]"
  Gain1/1 -> Cast/1  "Frame Time [us]"
  Gain/1 -> Cast1/1  "System Time [us]"
  Constant5/1 -> Bus Assignment/1
  Bus Assignment/1 -> System/1
  Cast/1 -> Bus Assignment/2
  Cast1/1 -> Bus Assignment/3

== system seldom_sim/Pilot Input/VelE_cmd ==
  dimensional_desired : Inport
  Constant : Constant  Value=172  OutDataTypeStr=single
  Constant2 : Constant  Value=Aircraft.Control.Limits.velocity_mps  OutDataTypeStr=single
  Constant3 : Constant  Value=1811  OutDataTypeStr=single
  Gain : Gain  Gain=-1
  remap : MATLAB Function  TreatAsAtomicUnit=on
  inceptor_ch_out : Outport
  wires:
  dimensional_desired/1 -> remap/1(raw_in)
  remap/1(norm_out) -> inceptor_ch_out/1
  Constant/1 -> remap/4(out_min)
  Constant3/1 -> remap/5(out_max)
  Constant2/1 -> remap/3(in_max), Gain/1
  Gain/1 -> remap/2(in_min)

== system seldom_sim/Pilot Input/VelN_cmd ==
  dimensional_desired : Inport
  Constant : Constant  Value=172  OutDataTypeStr=single
  Constant2 : Constant  Value=Aircraft.Control.Limits.velocity_mps  OutDataTypeStr=single
  Constant3 : Constant  Value=1811  OutDataTypeStr=single
  Gain : Gain  Gain=-1
  remap : MATLAB Function  TreatAsAtomicUnit=on
  inceptor_ch_out : Outport
  wires:
  Gain/1 -> remap/2(in_min)
  Constant2/1 -> Gain/1, remap/3(in_max)
  Constant3/1 -> remap/5(out_max)
  Constant/1 -> remap/4(out_min)
  remap/1(norm_out) -> inceptor_ch_out/1
  dimensional_desired/1 -> remap/1(raw_in)

== system seldom_sim/Pilot Input/VelU_cmd ==
  dimensional_desired : Inport
  Constant : Constant  Value=172  OutDataTypeStr=single
  Constant2 : Constant  Value=Aircraft.Control.Limits.velocity_mps  OutDataTypeStr=single
  Constant3 : Constant  Value=1811  OutDataTypeStr=single
  Gain : Gain  Gain=-1
  remap : MATLAB Function  TreatAsAtomicUnit=on
  inceptor_ch_out : Outport
  wires:
  dimensional_desired/1 -> remap/1(raw_in)
  remap/1(norm_out) -> inceptor_ch_out/1
  Constant/1 -> remap/4(out_min)
  Constant3/1 -> remap/5(out_max)
  Constant2/1 -> remap/3(in_max), Gain/1
  Gain/1 -> remap/2(in_min)

== system seldom_sim/Pilot Input/estop ==
  dimensional_desired : Inport
  Constant : Constant  Value=172  OutDataTypeStr=single
  Constant1 : Constant  Value=-1  OutDataTypeStr=single
  Constant2 : Constant  OutDataTypeStr=single
  Constant3 : Constant  Value=1811  OutDataTypeStr=single
  remap : MATLAB Function  TreatAsAtomicUnit=on
  inceptor_ch_out : Outport
  wires:
  dimensional_desired/1 -> remap/1(raw_in)
  remap/1(norm_out) -> inceptor_ch_out/1
  Constant/1 -> remap/4(out_min)
  Constant3/1 -> remap/5(out_max)
  Constant1/1 -> remap/2(in_min)
  Constant2/1 -> remap/3(in_max)

== system seldom_sim/Pilot Input/mode ==
  dimensional_desired : Inport
  Constant : Constant  Value=172  OutDataTypeStr=single
  Constant1 : Constant  Value=0  OutDataTypeStr=single
  Constant2 : Constant  Value=2  OutDataTypeStr=single
  Constant3 : Constant  Value=1811  OutDataTypeStr=single
  remap : MATLAB Function  TreatAsAtomicUnit=on
  inceptor_ch_out : Outport
  wires:
  Constant2/1 -> remap/3(in_max)
  Constant1/1 -> remap/2(in_min)
  Constant3/1 -> remap/5(out_max)
  Constant/1 -> remap/4(out_min)
  remap/1(norm_out) -> inceptor_ch_out/1
  dimensional_desired/1 -> remap/1(raw_in)

== system seldom_sim/Pilot Input/pitch_rate_cmd ==
  dimensional_desired : Inport
  Constant : Constant  Value=172  OutDataTypeStr=single
  Constant2 : Constant  Value=Aircraft.Control.Limits.angular_rate_rps  OutDataTypeStr=single
  Constant3 : Constant  Value=1811  OutDataTypeStr=single
  Gain : Gain  Gain=-1
  remap : MATLAB Function  TreatAsAtomicUnit=on
  inceptor_ch_out : Outport
  wires:
  dimensional_desired/1 -> remap/1(raw_in)
  remap/1(norm_out) -> inceptor_ch_out/1
  Constant/1 -> remap/4(out_min)
  Constant3/1 -> remap/5(out_max)
  Constant2/1 -> remap/3(in_max), Gain/1
  Gain/1 -> remap/2(in_min)

== system seldom_sim/Pilot Input/roll_rate_cmd ==
  dimensional_desired : Inport
  Constant : Constant  Value=172  OutDataTypeStr=single
  Constant2 : Constant  Value=Aircraft.Control.Limits.angular_rate_rps  OutDataTypeStr=single
  Constant3 : Constant  Value=1811  OutDataTypeStr=single
  Gain : Gain  Gain=-1
  remap : MATLAB Function  TreatAsAtomicUnit=on
  inceptor_ch_out : Outport
  wires:
  Gain/1 -> remap/2(in_min)
  Constant2/1 -> Gain/1, remap/3(in_max)
  Constant3/1 -> remap/5(out_max)
  Constant/1 -> remap/4(out_min)
  remap/1(norm_out) -> inceptor_ch_out/1
  dimensional_desired/1 -> remap/1(raw_in)

== system seldom_sim/Pilot Input/yaw_rate_cmd ==
  dimensional_desired : Inport
  Constant : Constant  Value=172  OutDataTypeStr=single
  Constant2 : Constant  Value=Aircraft.Control.Limits.angular_rate_rps  OutDataTypeStr=single
  Constant3 : Constant  Value=1811  OutDataTypeStr=single
  Gain : Gain  Gain=-1
  remap : MATLAB Function  TreatAsAtomicUnit=on
  inceptor_ch_out : Outport
  wires:
  Gain/1 -> remap/2(in_min)
  Constant2/1 -> Gain/1, remap/3(in_max)
  Constant3/1 -> remap/5(out_max)
  Constant/1 -> remap/4(out_min)
  remap/1(norm_out) -> inceptor_ch_out/1
  dimensional_desired/1 -> remap/1(raw_in)

== system seldom_sim/Vehicle/Forces and Moments ==
  note: Not touched for seldom, good as is.
  note: No idea what the aero for this vehicle would look like. Need to model this somehow in the future. Would also be dynamic derivatives for the Cl, Cm, and Cn that happend when the vehicle rotates.
  note: Overhauled for seldom.
  Dynamic Pressure [Pa] : Inport
  DCM_be : Inport  Port=2
  body_vel : Inport  Port=3
  Motor Cmds : Inport  Port=4
  Gravity [m/s/s] : Inport  Port=5
  Add : Sum  Inputs=+++
  Aerodynamic : Subsystem  Commented=on
  Demux3 : Demux  Outputs=2
  Gravitational : Subsystem
  Propulsive : Subsystem
  check for takeoff : Subsystem
  Fxyz [N] : Outport
  Mxyz [N-m] : Outport  Port=2
  wires:
  Add/1 -> Demux3/1
  Gravity [m/s/s]/1 -> Gravitational/1(Gravity [m/s/s])
  Motor Cmds/1 -> Propulsive/1(Motor Cmd)
  Demux3/1 -> Fxyz [N]/1
  Dynamic Pressure [Pa]/1 -> Aerodynamic/1(Dynamic Pressure)
  DCM_be/1 -> Gravitational/2(DCM_be)
  Demux3/2 -> Mxyz [N-m]/1
  body_vel/1 -> Aerodynamic/2(body_vel)
  Gravitational/1(Fxyz Mxyz) -> check for takeoff/2(FM_grav)
  check for takeoff/1(FM_prop_out) -> Add/1
  check for takeoff/2(FM_grav_out) -> Add/2
  check for takeoff/3(FM_aero_out) -> Add/3
  Aerodynamic/1(Fxyz Mxzy) -> check for takeoff/1(FM_aero)
  Propulsive/1(Fxyz Mxyz) -> check for takeoff/3(FM_prop)

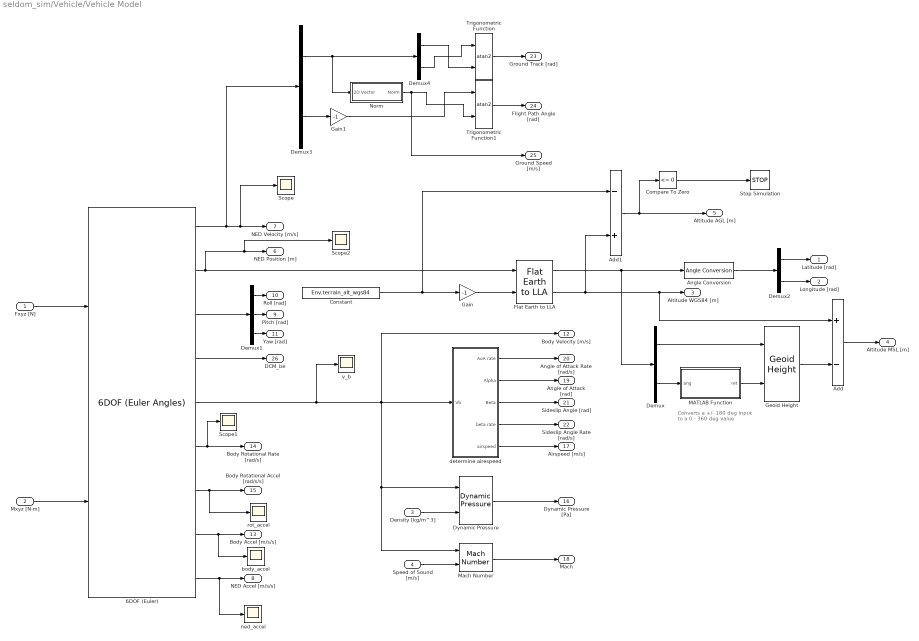
== system seldom_sim/Vehicle/Vehicle Model ==
  note: Converts a +/- 180 deg
      | input to a 0 - 360 deg value
  Fxyz [N] : Inport
  Mxyz [N-m] : Inport  Port=2
  Density [kg/m^3] : Inport  Port=3
  Speed of Sound [m/s] : Inport  Port=4
  6DOF (Euler) : shared6dof/6DOF (Euler Angles)  units=Metric (MKS)  mtype=Fixed  rep=Euler Angles  xme_0=InitCond.ned_pos_m  Vm_0=InitCond.body_vel_mps  eul_0=InitCond.euler_rad  pm_0=InitCond.body_rot_rate_radps  mass_0=Aircraft.Mass.mass_kg  mass_e=0.5  mass_f=2.0  inertia=Aircraft.Mass.inertia_kgm2  inertia_e=eye(3)  inertia_f=2*eye(3)  k_quat=1.0  vre_flag=on  abi_flag=on  aMode=0  xme_statename=''  Vm_statename=''  eul_statename=''  quat_statename=''  pm_statename=''  mass_statename=''
  Add : Sum  Inputs=+-
  Add1 : Sum  Inputs=-+
  Angle Conversion : aerolibconvert2/Angle Conversion  IU=deg  OU=rad
  Compare To Zero : simulink/Logic and Bit Operations/Compare To Zero  relop=<=  OutDataTypeStr=boolean
  Constant : Constant  Value=Env.terrain_alt_wgs84
  Demux : Demux  Outputs=2
  Demux1 : Demux  Outputs=3
  Demux2 : Demux  Outputs=2
  Demux3 : Demux  Outputs=[2 1]
  Demux4 : Demux  Outputs=2
  Dynamic Pressure : aerolibasang/Dynamic Pressure
  Flat Earth to LLA : aerolibtransform2/Flat Earth to LLA  units=Metric (MKS)  ptype=Earth (WGS84)  F=1/298.257223563  R=6378137  refPosPort=off  LL0=[rad2deg(InitCond.lat_rad) rad2deg(InitCond.lon_rad)]  psi=0
  Gain : Gain  Gain=-1
  Gain1 : Gain  Gain=-1
  Geoid Height : aerolibgravity2/Geoid Height  units=Metric (MKS)  gtype=EGM2008  datafile='geoidegm96grid'  dtype=double  action=Warning
  MATLAB Function : MATLAB Function  TreatAsAtomicUnit=on
  Mach Number : aerolibasang/Mach Number
  Norm : Subsystem
  Scope : Scope
  Scope1 : Scope
  Scope2 : Scope
  Stop Simulation : Stop
  Trigonometric Function : Trigonometry  Operator=atan2
  Trigonometric Function1 : Trigonometry  Operator=atan2
  body_accel : Scope
  determine airespeed : Subsystem
  ned_accel : Scope
  rot_accel : Scope
  v_b : Scope
  Latitude [rad] : Outport
  Longitude [rad] : Outport  Port=2
  Altitude WGS84 [m] : Outport  Port=3
  Altitude MSL [m] : Outport  Port=4
  Altitude AGL [m] : Outport  Port=5
  NED Position [m] : Outport  Port=6
  NED Velocity [m/s] : Outport  Port=7
  NED Accel [m/s/s] : Outport  Port=8
  Pitch [rad] : Outport  Port=9
  Roll [rad] : Outport  Port=10
  Yaw [rad] : Outport  Port=11
  Body Velocity [m/s] : Outport  Port=12
  Body Accel [m/s/s] : Outport  Port=13
  Body Rotational Rate [rad/s] : Outport  Port=14
  Body Rotational Accel [rad/s/s] : Outport  Port=15
  Dynamic Pressure [Pa] : Outport  Port=16
  Airspeed [m/s] : Outport  Port=17
  Mach : Outport  Port=18
  Angle of Attack [rad] : Outport  Port=19
  Angle of Attack Rate [rad/s] : Outport  Port=20
  Sideslip Angle [rad] : Outport  Port=21
  Sideslip Angle Rate [rad/s] : Outport  Port=22
  Ground Track [rad] : Outport  Port=23
  Flight Path Angle [rad] : Outport  Port=24
  Ground Speed [m/s] : Outport  Port=25
  DCM_be : Outport  Port=26
  wires:
  Fxyz [N]/1 -> 6DOF (Euler)/1
  Mxyz [N-m]/1 -> 6DOF (Euler)/2
  6DOF (Euler)/5 -> v_b/1, determine airespeed/1(Vb), Dynamic Pressure/1, Mach Number/1, Body Velocity [m/s]/1
  Flat Earth to LLA/1 -> Demux/1, Angle Conversion/1
  Flat Earth to LLA/2 -> Add1/2, Add/1, Altitude WGS84 [m]/1
  Demux/2 -> MATLAB Function/1(ang)
  Demux/1 -> Geoid Height/1
  Density [kg/m^3]/1 -> Dynamic Pressure/2
  Angle Conversion/1 -> Demux2/1
  6DOF (Euler)/4 -> DCM_be/1
  Demux1/1 -> Roll [rad]/1
  6DOF (Euler)/3 -> Demux1/1
  Demux1/2 -> Pitch [rad]/1
  Demux1/3 -> Yaw [rad]/1
  Dynamic Pressure/1 -> Dynamic Pressure [Pa]/1
  Add/1 -> Altitude MSL [m]/1
  Gain/1 -> Flat Earth to LLA/2
  Demux2/2 -> Longitude [rad]/1
  Demux2/1 -> Latitude [rad]/1
  6DOF (Euler)/2 -> Scope2/1, NED Position [m]/1, Flat Earth to LLA/1
  6DOF (Euler)/6 -> Scope1/1, Body Rotational Rate [rad/s]/1
  6DOF (Euler)/7 -> rot_accel/1, Body Rotational Accel [rad/s/s]/1
  6DOF (Euler)/1 -> Demux3/1, Scope/1, NED Velocity [m/s]/1
  MATLAB Function/1(ret) -> Geoid Height/2
  Demux3/1 -> Norm/1(2D Vector), Demux4/1
  Trigonometric Function/1 -> Ground Track [rad]/1
  Demux3/2 -> Gain1/1
  Gain1/1 -> Trigonometric Function1/1
  Norm/1(Norm) -> Ground Speed [m/s]/1, Trigonometric Function1/2
  Trigonometric Function1/1 -> Flight Path Angle [rad]/1
  6DOF (Euler)/9 -> ned_accel/1, NED Accel [m/s/s]/1
  Speed of Sound [m/s]/1 -> Mach Number/2
  Mach Number/1 -> Mach/1
  Constant/1 -> Add1/1, Gain/1
  Add1/1 -> Compare To Zero/1, Altitude AGL [m]/1
  Compare To Zero/1 -> Stop Simulation/1
  Demux4/1 -> Trigonometric Function/2
  Demux4/2 -> Trigonometric Function/1
  6DOF (Euler)/8 -> body_accel/1, Body Accel [m/s/s]/1
  determine airespeed/1(AoA rate) -> Angle of Attack Rate [rad/s]/1
  determine airespeed/2(Alpha) -> Angle of Attack [rad]/1
  determine airespeed/3(Beta) -> Sideslip Angle [rad]/1
  determine airespeed/4(beta rate) -> Sideslip Angle Rate [rad/s]/1
  determine airespeed/5(airspeed) -> Airspeed [m/s]/1
  Geoid Height/1 -> Add/2

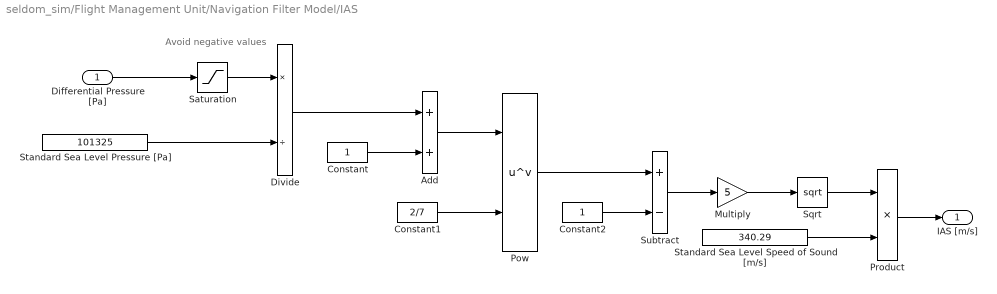
== system seldom_sim/Flight Management Unit/Navigation Filter Model/IAS ==
  note: Avoid negative values
  Differential Pressure [Pa] : Inport
  Add : Sum
  Constant : Constant  OutDataTypeStr=double
  Constant1 : Constant  Value=2/7  OutDataTypeStr=double
  Constant2 : Constant  OutDataTypeStr=double
  Divide : Product  Inputs=*/
  Multiply : Gain  Gain=5
  Pow : Math  Operator=pow  RndMeth=Zero
  Product : Product
  Saturation : Saturate  UpperLimit=inf  LowerLimit=0
  Sqrt : Sqrt
  Standard Sea Level Pressure [Pa] : Constant  Value=101325  OutDataTypeStr=double
  Standard Sea Level Speed of Sound [m/s] : Constant  Value=340.29  OutDataTypeStr=double
  Subtract : Sum  Inputs=+-
  IAS [m/s] : Outport
  wires:
  Differential Pressure [Pa]/1 -> Saturation/1
  Saturation/1 -> Divide/1
  Standard Sea Level Pressure [Pa]/1 -> Divide/2
  Divide/1 -> Add/1
  Constant/1 -> Add/2
  Constant1/1 -> Pow/2
  Add/1 -> Pow/1
  Pow/1 -> Subtract/1
  Constant2/1 -> Subtract/2
  Subtract/1 -> Multiply/1
  Multiply/1 -> Sqrt/1
  Sqrt/1 -> Product/1
  Product/1 -> IAS [m/s]/1
  Standard Sea Level Speed of Sound [m/s]/1 -> Product/2

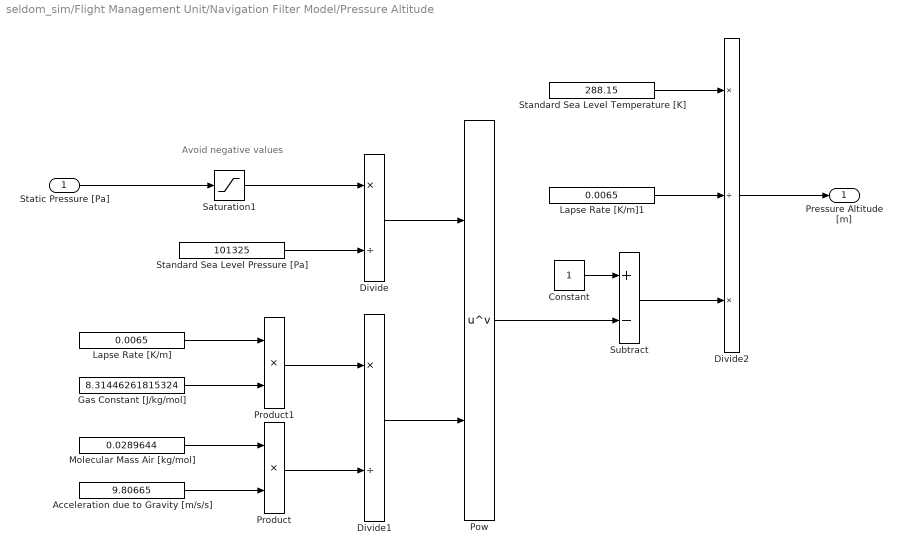
== system seldom_sim/Flight Management Unit/Navigation Filter Model/Pressure Altitude ==
  note: Avoid negative values
  Static Pressure [Pa] : Inport
  Acceleration due to Gravity [m/s/s] : Constant  Value=9.80665  OutDataTypeStr=double
  Constant : Constant  OutDataTypeStr=double
  Divide : Product  Inputs=*/
  Divide1 : Product  Inputs=*/
  Divide2 : Product  Inputs=*/*
  Gas Constant [J/kg/mol] : Constant  Value=8.31446261815324  OutDataTypeStr=double
  Lapse Rate [K/m] : Constant  Value=0.0065  OutDataTypeStr=double
  Lapse Rate [K/m]1 : Constant  Value=0.0065  OutDataTypeStr=double
  Molecular Mass Air [kg/mol] : Constant  Value=0.0289644  OutDataTypeStr=double
  Pow : Math  Operator=pow  RndMeth=Zero
  Product : Product
  Product1 : Product
  Saturation1 : Saturate  UpperLimit=inf  LowerLimit=0
  Standard Sea Level Pressure [Pa] : Constant  Value=101325  OutDataTypeStr=double
  Standard Sea Level Temperature [K] : Constant  Value=288.15  OutDataTypeStr=double
  Subtract : Sum  Inputs=+-
  Pressure Altitude [m] : Outport
  wires:
  Static Pressure [Pa]/1 -> Saturation1/1
  Saturation1/1 -> Divide/1
  Standard Sea Level Pressure [Pa]/1 -> Divide/2
  Divide/1 -> Pow/1
  Product1/1 -> Divide1/1
  Product/1 -> Divide1/2
  Molecular Mass Air [kg/mol]/1 -> Product/1
  Acceleration due to Gravity [m/s/s]/1 -> Product/2
  Gas Constant [J/kg/mol]/1 -> Product1/2
  Lapse Rate [K/m]/1 -> Product1/1
  Divide1/1 -> Pow/2
  Pow/1 -> Subtract/2
  Constant/1 -> Subtract/1
  Subtract/1 -> Divide2/3
  Divide2/1 -> Pressure Altitude [m]/1
  Lapse Rate [K/m]1/1 -> Divide2/2
  Standard Sea Level Temperature [K]/1 -> Divide2/1

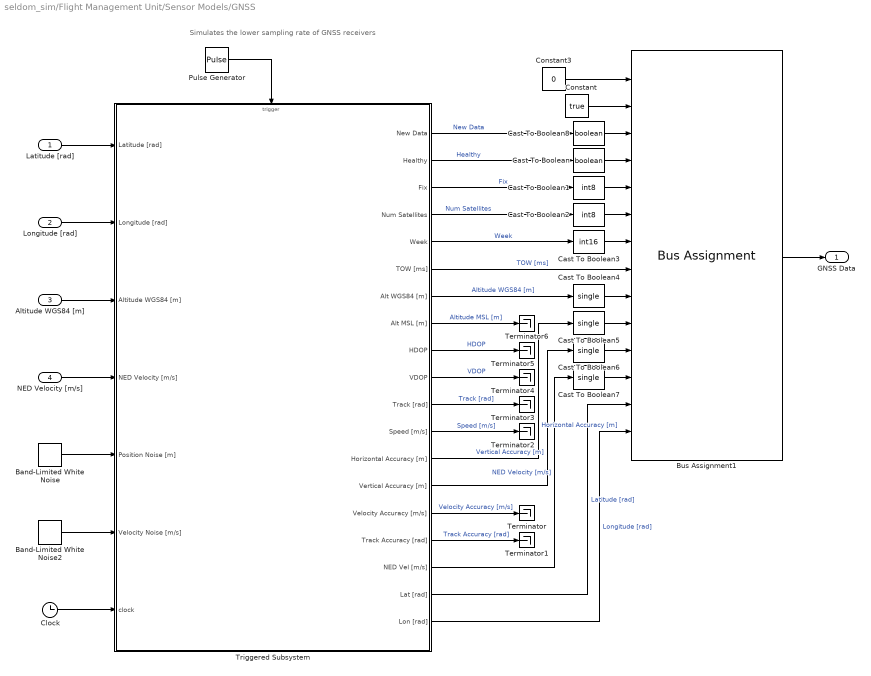
== system seldom_sim/Flight Management Unit/Sensor Models/GNSS ==
  note: Simulates the lower sampling rate of GNSS receivers
  Latitude [rad] : Inport
  "Longitude [rad] " : Inport  Port=2
  Altitude WGS84 [m] : Inport  Port=3
  NED Velocity [m/s] : Inport  Port=4
  Band-Limited White Noise : simulink/Sources/Band-Limited White Noise  Cov=[Aircraft.Sensors.Gnss.horz_accuracy_m Aircraft.Sensors.Gnss.horz_accuracy_m Aircraft.Sensors.Gnss.vert_accuracy_m]  Ts=0.1  seed=[23341]
  Band-Limited White Noise2 : simulink/Sources/Band-Limited White Noise  Cov=Aircraft.Sensors.Gnss.vel_accuracy_mps * ones(3, 1)  Ts=0.1  seed=[23341]
  Bus Assignment1 : BusAssignment  AssignedSignals=installed,new_data,healthy,fix,num_sats,week,gps_tow_ms,alt_wgs84_m,horz_acc_m,vert_acc_m,ned_vel_mps,lat_rad,lon_rad
  Cast To Boolean : DataTypeConversion  OutDataTypeStr=boolean  SaturateOnIntegerOverflow=off  RndMeth=Floor
  Cast To Boolean1 : DataTypeConversion  OutDataTypeStr=int8  SaturateOnIntegerOverflow=off  RndMeth=Floor
  Cast To Boolean2 : DataTypeConversion  OutDataTypeStr=int8  SaturateOnIntegerOverflow=off  RndMeth=Floor
  Cast To Boolean3 : DataTypeConversion  OutDataTypeStr=int16  SaturateOnIntegerOverflow=off  RndMeth=Floor
  Cast To Boolean{4..7} (4 alike) : DataTypeConversion  OutDataTypeStr=single  SaturateOnIntegerOverflow=off  RndMeth=Floor
  Cast To Boolean8 : DataTypeConversion  OutDataTypeStr=boolean  SaturateOnIntegerOverflow=off  RndMeth=Floor
  Clock : Clock
  Constant : Constant  Value=true
  Constant3 : Constant  Value=0  OutDataTypeStr=Bus: GnssData
  Pulse Generator : DiscretePulseGenerator  PulseType=Time based  Period=1/Aircraft.Sensors.Gnss.sample_rate_hz  PulseWidth=5
  Terminator{,1..6} (7 alike) : Terminator
  Triggered Subsystem : Subsystem  TreatAsAtomicUnit=on
  GNSS Data : Outport
  wires:
  Bus Assignment1/1 -> GNSS Data/1
  NED Velocity [m/s]/1 -> Triggered Subsystem/4(NED Velocity [m/s])
  Altitude WGS84 [m]/1 -> Triggered Subsystem/3(Altitude WGS84 [m])
  "Longitude [rad] "/1 -> Triggered Subsystem/2("Longitude [rad] ")
  Clock/1 -> Triggered Subsystem/7(clock)
  Band-Limited White Noise/1 -> Triggered Subsystem/5(Position Noise [m])
  Pulse Generator/1 -> Triggered Subsystem/Trigger
  Band-Limited White Noise2/1 -> Triggered Subsystem/6(Velocity Noise [m/s])
  Latitude [rad]/1 -> Triggered Subsystem/1(Latitude [rad])
  Triggered Subsystem/1(New Data) -> Cast To Boolean8/1  "New Data"
  Triggered Subsystem/2(Healthy) -> Cast To Boolean/1  "Healthy"
  Triggered Subsystem/3(Fix) -> Cast To Boolean1/1  "Fix"
  Triggered Subsystem/4(Num Satellites) -> Cast To Boolean2/1  "Num Satellites"
  Triggered Subsystem/5(Week) -> Cast To Boolean3/1  "Week"
  Triggered Subsystem/6(TOW [ms]) -> Bus Assignment1/8  "TOW [ms]"
  Triggered Subsystem/7(Alt WGS84 [m]) -> Cast To Boolean4/1  "Altitude WGS84 [m]"
  Triggered Subsystem/8(Alt MSL [m]) -> Terminator6/1  "Altitude MSL [m]"
  Triggered Subsystem/9(HDOP) -> Terminator5/1  "HDOP"
  Triggered Subsystem/10(VDOP) -> Terminator4/1  "VDOP"
  Triggered Subsystem/11(Track [rad]) -> Terminator3/1  "Track [rad]"
  Triggered Subsystem/12(Speed [m/s]) -> Terminator2/1  "Speed [m/s]"
  Triggered Subsystem/13(Horizontal Accuracy [m]) -> Cast To Boolean5/1  "Horizontal Accuracy [m]"
  Triggered Subsystem/14(Vertical Accuracy [m]) -> Cast To Boolean6/1  "Vertical Accuracy [m]"
  Triggered Subsystem/15(Velocity Accuracy [m/s]) -> Terminator/1  "Velocity Accuracy [m/s]"
  Triggered Subsystem/16(Track Accuracy [rad]) -> Terminator1/1  "Track Accuracy [rad]"
  Triggered Subsystem/17(NED Vel [m/s]) -> Cast To Boolean7/1  "NED Velocity [m/s]"
  Triggered Subsystem/18(Lat [rad]) -> Bus Assignment1/13  "Latitude [rad]"
  Triggered Subsystem/19(Lon [rad]) -> Bus Assignment1/14  "Longitude [rad]"
  Constant3/1 -> Bus Assignment1/1
  Constant/1 -> Bus Assignment1/2
  Cast To Boolean/1 -> Bus Assignment1/4
  Cast To Boolean1/1 -> Bus Assignment1/5
  Cast To Boolean2/1 -> Bus Assignment1/6
  Cast To Boolean3/1 -> Bus Assignment1/7
  Cast To Boolean4/1 -> Bus Assignment1/9
  Cast To Boolean5/1 -> Bus Assignment1/10
  Cast To Boolean6/1 -> Bus Assignment1/11
  Cast To Boolean7/1 -> Bus Assignment1/12
  Cast To Boolean8/1 -> Bus Assignment1/3
